simulink model "A_Justo_SCHFV_slx_UFHDV_Design_LinNoGS"  (R2019a)
settings: Solver=VariableStepAuto  StartTime=0.0  StopTime=tfinal  MaxStep=maxstepsize  RelTol=1e-3  EnableMultiTasking=on
model workspace (MAT data in the model file):
  sims_v_H = Simulink.Parameter
  sims_v_H.DataType = 'auto'
  sims_v_H.Dimensions = [0 0]
values from neighbouring files (symbols this model uses):
  aini = 0    [A_Justo_SCHFV_m_UFHDV_Design.m]
  eta = sum(normrnd(IDM_t,IDM_ts,1,n))    [A_Justo_SCHFV_m_Control_Sensitivity.m]    (also in A_Justo_SCHFV_m_UFHDV_Design.m; TransferFunctionPROP.m = IDM_T(acc1+n1,acc1+n1))
  hini = 1.01*IDM_H0    [A_Justo_SCHFV_m_UFHDV_Design.m]
  IDM_Amax = IDM_Amax(acc1+n1,acc1+n1)    [TransferFunctionPROP.m]
  IDM_Bmax = IDM_Bmax(acc1+n1,acc1+n1)    [TransferFunctionPROP.m]
  IDM_Delta = IDM_Delta(acc1+n1)    [TransferFunctionPROP.m]
  IDM_H0 = IDM_H0(acc1+n1)    [TransferFunctionPROP.m]
  IDM_T = normrnd(IDM_t,IDM_ts)    [A_Justo_SCHFV_m_Control_Sensitivity.m]    (also in A_Justo_SCHFV_m_Track.m = IDM_Tind; A_Justo_SCHFV_m_UFHDV_Design.m; TransferFunctionPROP.m = IDM_T(acc1+n1,acc1+n1))
  IDM_V0 = IDM_V0(acc1+n1)    [TransferFunctionPROP.m]
  K = [k1 k2 k3 k4 k5]    [A_Justo_SCHFV_m_Control_Sensitivity.m]    (also in A_Justo_SCHFV_m_UFHDV_Design.m)
  kz = K(6)    [A_Justo_SCHFV_m_Control_Sensitivity.m]    (also in A_Justo_SCHFV_m_UFHDV_Design.m)
  Lini = Lind    [A_Justo_SCHFV_m_Track.m]    (also in A_Justo_SCHFV_m_UFHDV_Design.m = sum(normrnd(l,ls,1,n)))
  Tau_A = normrnd(tau,taus)    [A_Justo_SCHFV_m_Control_Sensitivity.m]    (also in A_Justo_SCHFV_m_UFHDV_Design.m; TransferFunctionPROP.m = Tau(acc1,acc1))
  Tau_H = normrnd(tau,taus)    [A_Justo_SCHFV_m_Control_Sensitivity.m]    (also in A_Justo_SCHFV_m_UFHDV_Design.m; TransferFunctionPROP.m = Tau(acc1+n1,acc1+n1))
  v_r_0 = 30/3.6    (= 8.33333333333)    [A_Justo_SCHFV_m_Control_Sensitivity.m]    (also in A_Justo_SCHFV_m_Track.m = 5.55555555556; A_Justo_SCHFV_m_UFHDV_Design.m = 2.77777777778)
  vini = 0    [A_Justo_SCHFV_m_UFHDV_Design.m]
  zini = 0    [A_Justo_SCHFV_m_UFHDV_Design.m]
settings Model: Creator=arnaudoria  LastModifiedBy=Sander
settings DataIOCC: LimitDataPoints=on  ReturnWorkspaceOutputs=off
settings OptimizationCC: LifeSpan=inf
settings DebuggingCC: AllowSymbolicDim=off  SFUnexpectedBacktrackingDiag=warning  SFNoUnconditionalDefaultTransitionDiag=warning  SFExecutionAtInitializationDiag=none  ArithmeticOperatorsInVariantConditions=warning
settings ModelReferenceCC: PropagateSignalLabelsOutOfModel=off
settings SFSimCC: SimUseLocalCustomCode=off
settings RTWCC: RTWUseLocalCustomCode=off
settings CodeAppCC: StateflowObjectComments=on
settings GRTTargetCC: TargetLangStandard=C89/C90 (ANSI)
settings ConfigComp: CovMetricSettings=dw  CovHtmlReporting=on  CovSaveCumulativeToWorkspaceVar=on  CovSaveSingleToWorkspaceVar=on  CovExternalEMLEnable=off

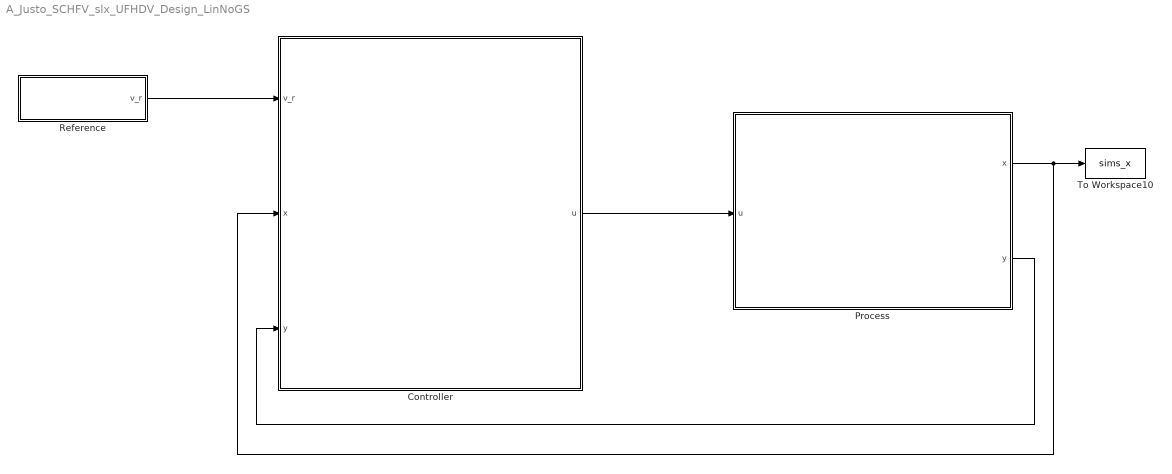
== system A_Justo_SCHFV_slx_UFHDV_Design_LinNoGS ==
  Controller : Subsystem
  Process : Subsystem
  Reference : Subsystem
  To Workspace10 : ToWorkspace  VariableName=sims_x  SampleTime=-1
  wires:
  Controller/1(u) -> Process/1(u)
  Process/2(y) -> Controller/3(y)
  Process/1(x) -> Controller/2(x), To Workspace10/1
  Reference/1(v_r) -> Controller/1(v_r)

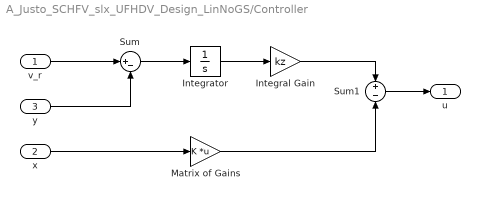
== system A_Justo_SCHFV_slx_UFHDV_Design_LinNoGS/Controller ==
  v_r : Inport
  x : Inport  Port=2
  y : Inport  Port=3
  Integral Gain : Gain  Gain=kz
  Integrator : Integrator  InitialCondition=zini
  Matrix of Gains : Gain  Gain=K  Multiplication=Matrix(K*u)
  Sum : Sum  Inputs=|+-
  Sum1 : Sum  Inputs=+|-
  u : Outport
  wires:
  Sum1/1 -> u/1
  Integrator/1 -> Integral Gain/1
  Sum/1 -> Integrator/1
  Integral Gain/1 -> Sum1/1
  v_r/1 -> Sum/1
  Matrix of Gains/1 -> Sum1/2
  y/1 -> Sum/2
  x/1 -> Matrix of Gains/1

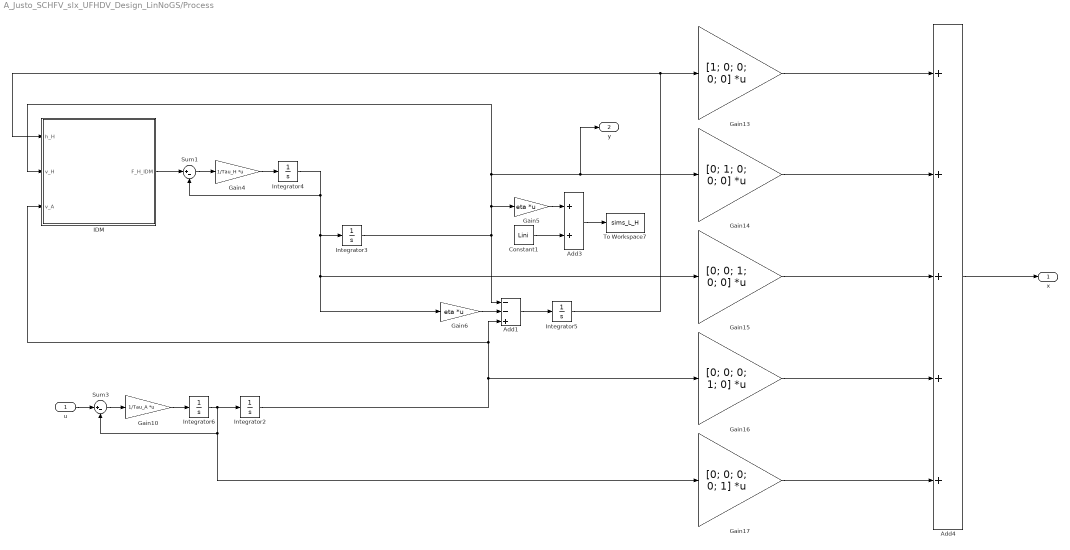
== system A_Justo_SCHFV_slx_UFHDV_Design_LinNoGS/Process ==
  u : Inport
  Add1 : Sum  Inputs=--+
  Add3 : Sum
  Add4 : Sum  Inputs=+++++
  Constant1 : Constant  Value=Lini
  Gain10 : Gain  Gain=1/Tau_A  Multiplication=Matrix(K*u)
  Gain13 : Gain  Gain=[1; 0; 0; 0; 0]  Multiplication=Matrix(K*u)
  Gain14 : Gain  Gain=[0; 1; 0; 0; 0]  Multiplication=Matrix(K*u)
  Gain15 : Gain  Gain=[0; 0; 1; 0; 0]  Multiplication=Matrix(K*u)
  Gain16 : Gain  Gain=[0; 0; 0; 1; 0]  Multiplication=Matrix(K*u)
  Gain17 : Gain  Gain=[0; 0; 0; 0; 1]  Multiplication=Matrix(K*u)
  Gain4 : Gain  Gain=1/Tau_H  Multiplication=Matrix(K*u)
  Gain5 : Gain  Gain=eta  Multiplication=Matrix(K*u)
  Gain6 : Gain  Gain=eta  Multiplication=Matrix(K*u)
  IDM : Subsystem
  Integrator2 : Integrator  InitialCondition=vini  WrappedStateUpperValue=2*pi  WrappedStateLowerValue=0
  Integrator3 : Integrator  InitialCondition=vini  WrappedStateUpperValue=2*pi  WrappedStateLowerValue=0
  Integrator4 : Integrator  InitialCondition=aini  WrappedStateUpperValue=2*pi  WrappedStateLowerValue=0
  Integrator5 : Integrator  InitialCondition=hini  WrappedStateUpperValue=2*pi  WrappedStateLowerValue=0
  Integrator6 : Integrator  InitialCondition=aini  WrappedStateUpperValue=2*pi  WrappedStateLowerValue=0
  Sum1 : Sum  Inputs=|+-
  Sum3 : Sum  Inputs=|+-
  To Workspace7 : ToWorkspace  VariableName=sims_L_H  SampleTime=-1
  x : Outport
  y : Outport  Port=2
  wires:
  u/1 -> Sum3/1
  Add1/1 -> Integrator5/1
  Gain5/1 -> Add3/1
  Integrator6/1 -> Gain17/1, Sum3/2, Integrator2/1
  Integrator4/1 -> Integrator3/1, Gain6/1, Gain15/1, Sum1/2
  Constant1/1 -> Add3/2
  Add3/1 -> To Workspace7/1
  Sum3/1 -> Gain10/1
  Gain10/1 -> Integrator6/1
  Integrator5/1 -> IDM/1(h_H), Gain13/1
  Sum1/1 -> Gain4/1
  Gain4/1 -> Integrator4/1
  Integrator3/1 -> Add1/1, IDM/2(v_H), Gain14/1, y/1, Gain5/1
  Gain17/1 -> Add4/5
  Gain16/1 -> Add4/4
  Gain15/1 -> Add4/3
  Gain14/1 -> Add4/2
  Gain13/1 -> Add4/1
  Add4/1 -> x/1
  Gain6/1 -> Add1/2
  IDM/1(F_H_IDM) -> Sum1/1
  Integrator2/1 -> Gain16/1, Add1/3, IDM/3(v_A)

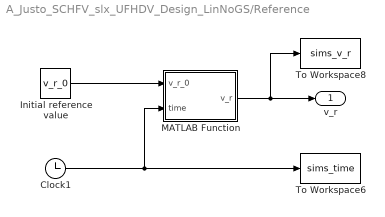
== system A_Justo_SCHFV_slx_UFHDV_Design_LinNoGS/Reference ==
  Clock1 : Clock
  Initial reference value : Constant  Value=v_r_0
  MATLAB Function : MATLAB Function  TreatAsAtomicUnit=on
  To Workspace6 : ToWorkspace  VariableName=sims_time  SampleTime=-1
  To Workspace8 : ToWorkspace  VariableName=sims_v_r  SampleTime=-1
  v_r : Outport
  wires:
  Clock1/1 -> To Workspace6/1, MATLAB Function/2(time)
  MATLAB Function/1(v_r) -> v_r/1, To Workspace8/1
  Initial reference value/1 -> MATLAB Function/1(v_r_0)

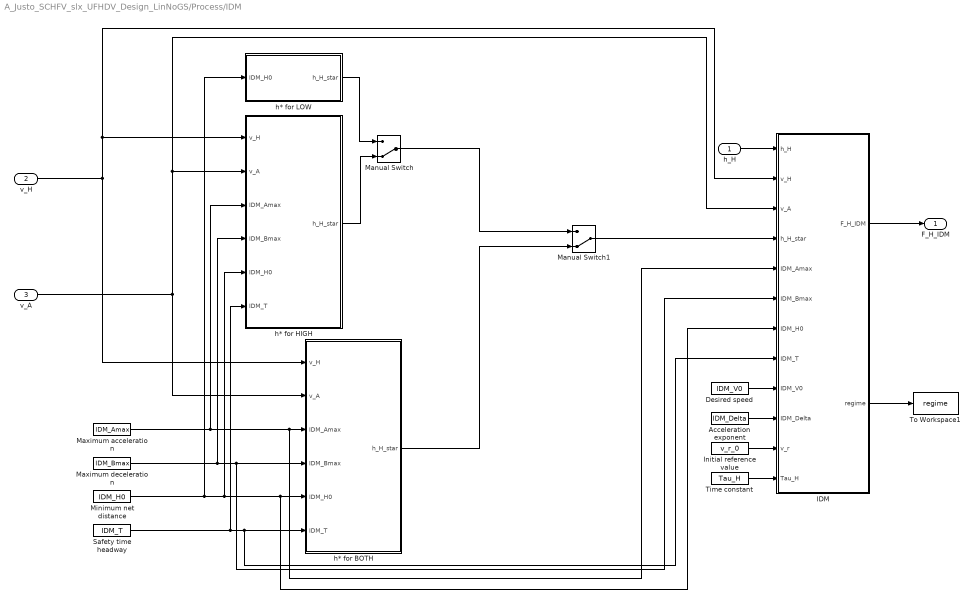
== system A_Justo_SCHFV_slx_UFHDV_Design_LinNoGS/Process/IDM ==
  h_H : Inport
  v_H : Inport  Port=2
  v_A : Inport  Port=3
  Acceleration exponent : Constant  Value=IDM_Delta
  Desired speed : Constant  Value=IDM_V0
  IDM : MATLAB Function  TreatAsAtomicUnit=on
  Initial reference value : Constant  Value=v_r_0
  Manual Switch : ManualSwitch  CurrentSetting=0
  Manual Switch1 : ManualSwitch  CurrentSetting=0
  Maximum acceleration : Constant  Value=IDM_Amax
  Maximum deceleration : Constant  Value=IDM_Bmax
  Minimum net distance : Constant  Value=IDM_H0
  Safety time headway : Constant  Value=IDM_T
  Time constant : Constant  Value=Tau_H
  To Workspace1 : ToWorkspace  VariableName=regime  SampleTime=-1
  h* for BOTH : MATLAB Function  TreatAsAtomicUnit=on
  h* for HIGH : MATLAB Function  TreatAsAtomicUnit=on
  h* for LOW : MATLAB Function  TreatAsAtomicUnit=on
  F_H_IDM : Outport
  wires:
  Acceleration exponent/1 -> IDM/10(IDM_Delta)
  Desired speed/1 -> IDM/9(IDM_V0)
  IDM/2(regime) -> To Workspace1/1
  IDM/1(F_H_IDM) -> F_H_IDM/1
  Minimum net distance/1 -> h* for HIGH/5(IDM_H0), h* for BOTH/5(IDM_H0), IDM/7(IDM_H0), h* for LOW/1(IDM_H0)
  Maximum acceleration/1 -> h* for HIGH/3(IDM_Amax), h* for BOTH/3(IDM_Amax), IDM/5(IDM_Amax)
  Safety time headway/1 -> h* for HIGH/6(IDM_T), IDM/8(IDM_T), h* for BOTH/6(IDM_T)
  Maximum deceleration/1 -> h* for HIGH/4(IDM_Bmax), IDM/6(IDM_Bmax), h* for BOTH/4(IDM_Bmax)
  h_H/1 -> IDM/1(h_H)
  h* for LOW/1(h_H_star) -> Manual Switch/1
  h* for HIGH/1(h_H_star) -> Manual Switch/2
  Manual Switch/1 -> Manual Switch1/1
  h* for BOTH/1(h_H_star) -> Manual Switch1/2
  Manual Switch1/1 -> IDM/4(h_H_star)
  v_H/1 -> h* for HIGH/1(v_H), IDM/2(v_H), h* for BOTH/1(v_H)
  v_A/1 -> IDM/3(v_A), h* for HIGH/2(v_A), h* for BOTH/2(v_A)
  Initial reference value/1 -> IDM/11(v_r)
  Time constant/1 -> IDM/12(Tau_H)

== matlab function A_Justo_SCHFV_slx_UFHDV_Design_LinNoGS/Reference/MATLAB Function ==
  data: v_r_0 input; v_r output; time input
function v_r = fcn(v_r_0, time)
v_r=v_r_0;
% if time < 50
%     v_r = v_r_0;
% elseif time >=50 && time <100
%     v_r = 2*v_r_0;
% elseif time >=100 && time <150
%     v_r = 3*v_r_0;
% elseif time >=150 && time <200
%     v_r = 4*v_r_0;
% else
%     v_r = 5*v_r_0;
% end

== matlab function A_Justo_SCHFV_slx_UFHDV_Design_LinNoGS/Process/IDM/h* for HIGH ==
  data: v_H input; h_H_star output; v_A input; IDM_Amax input; IDM_Bmax input; IDM_H0 input; IDM_T input
function h_H_star = fcn(v_H,v_A,IDM_Amax,IDM_Bmax,IDM_H0,IDM_T)
h_H_star = IDM_H0 + IDM_T*v_H + v_H*(v_H-v_A)/(2*sqrt(IDM_Amax*IDM_Bmax));
end

== matlab function A_Justo_SCHFV_slx_UFHDV_Design_LinNoGS/Process/IDM/h* for LOW ==
  data: h_H_star output; IDM_H0 input
function h_H_star = fcn(IDM_H0)
h_H_star = IDM_H0;
end

== matlab function A_Justo_SCHFV_slx_UFHDV_Design_LinNoGS/Process/IDM/h* for BOTH ==
  data: v_H input; h_H_star output; v_A input; IDM_Amax input; IDM_Bmax input; IDM_H0 input; IDM_T input
function h_H_star = fcn(v_H,v_A,IDM_Amax,IDM_Bmax,IDM_H0,IDM_T)
h_H_star = IDM_H0 + ...
    max( 0, IDM_T*v_H + v_H*(v_H-v_A)/(2*sqrt(IDM_Amax*IDM_Bmax)) );
end

== matlab function A_Justo_SCHFV_slx_UFHDV_Design_LinNoGS/Process/IDM/IDM ==
  data: h_H input; v_H input; v_A input; h_H_star input; IDM_Amax input; IDM_Bmax input; IDM_H0 input; IDM_T input; IDM_V0 input; IDM_Delta input; F_H_IDM output; regime output; v_r input; Tau_H input
function [F_H_IDM,regime] = fcn(h_H,v_H,v_A,h_H_star,IDM_Amax,IDM_Bmax,IDM_H0,IDM_T,IDM_V0,IDM_Delta,v_r,Tau_H)
if h_H_star == IDM_H0
    regime=0;
    A31 = 2*IDM_Amax/(Tau_H*IDM_H0)*(1-(v_r/IDM_V0)^IDM_Delta)^(3/2);
    A32 = -IDM_Amax/Tau_H*(IDM_Delta*v_r^(IDM_Delta-1)/IDM_V0^IDM_Delta);
    A34 = 0;
else
    regime=1;
    A31 = 2*IDM_Amax/(Tau_H*(IDM_H0+v_r*IDM_T))*(1-(v_r/IDM_V0)^IDM_Delta)^(3/2);
    A32 = -IDM_Amax/Tau_H*(IDM_Delta*v_r^(IDM_Delta-1)/IDM_V0^IDM_Delta+(v_r+2*IDM_T*sqrt(IDM_Amax*IDM_Bmax))/((IDM_H0+v_r*IDM_T)*sqrt(IDM_Amax*IDM_Bmax))*(1-(v_r/IDM_V0)^IDM_Delta));
    A34 = IDM_Amax*v_r/(Tau_H*((IDM_H0+v_r*IDM_T)*sqrt(IDM_Amax*IDM_Bmax)))*(1-(v_r/IDM_V0)^IDM_Delta);
end
F_H_IDM = A31*h_H + A32*v_H + A34*v_A;
end
